simulink model "Kenh_B"  (R2017b)
settings: Solver=FixedStepDiscrete  StartTime=0.0  StopTime=inf  FixedStep=0.0005  RelTol=1e-3  EnableMultiTasking=on
libraries: arduinolib x4, simulink x3
settings Model: SimulationMode=external  ExtModeTrigDuration=2  Creator=Admin  LastModifiedBy=Admin
settings SolverCC: AutoInsertRateTranBlk=on
settings DataIOCC: LimitDataPoints=on
settings OptimizationCC: PassReuseOutputArgsAs=Individual arguments  MaxStackSize=64
settings DebuggingCC: ParameterTunabilityLossMsg=error  AllowSymbolicDim=off  SFUnexpectedBacktrackingDiag=warning  SFNoUnconditionalDefaultTransitionDiag=warning  SFExecutionAtInitializationDiag=none
settings HardwareCC: ProdBitPerInt=16  ProdBitPerPointer=16  ProdBitPerSizeT=16  ProdBitPerPtrDiffT=16  ProdLargestAtomicFloat=None  ProdWordSize=8  ProdHWDeviceType=Atmel->AVR
settings SFSimCC: MATLABDynamicMemAlloc=off
settings RTWCC: SystemTargetFile=ert.tlc  HardwareBoard=Arduino Uno  TLCOptions=-aInlineSetEventsForThisBaseRateFcn=TLC_FALSE -aSuppressMultiTaskScheduler=TLC_FALSE -aRateBasedStepFcn=1  TemplateMakefile=ert_default_tmf  GenerateReport=on  Toolchain=Arduino AVR  BuildConfiguration=Faster Runs  IncludeHyperlinkInReport=on  LaunchReport=on  GenerateTraceInfo=on  GenerateTraceReport=on  GenerateTraceReportSl=on  GenerateTraceReportSf=on  GenerateTraceReportEml=on
settings CodeAppCC: ForceParamTrailComments=on  IgnoreCustomStorageClasses=off  OperatorAnnotations=on  SimulinkDataObjDesc=on  SFDataObjDesc=on  InsertBlockDesc=on
settings ERTTargetCC: SupportContinuousTime=on  SupportVariableSizeSignals=on  ExtMode=on  ExtModeMexArgs='127.0.0.1' 0 17725
settings ConfigComp: CovMetricSettings=dw  CovHtmlReporting=on  CovSaveCumulativeToWorkspaceVar=on  CovSaveSingleToWorkspaceVar=on  CovShowResultsExplorer=off  CovExternalEMLEnable=off  CovSFcnEnable=off

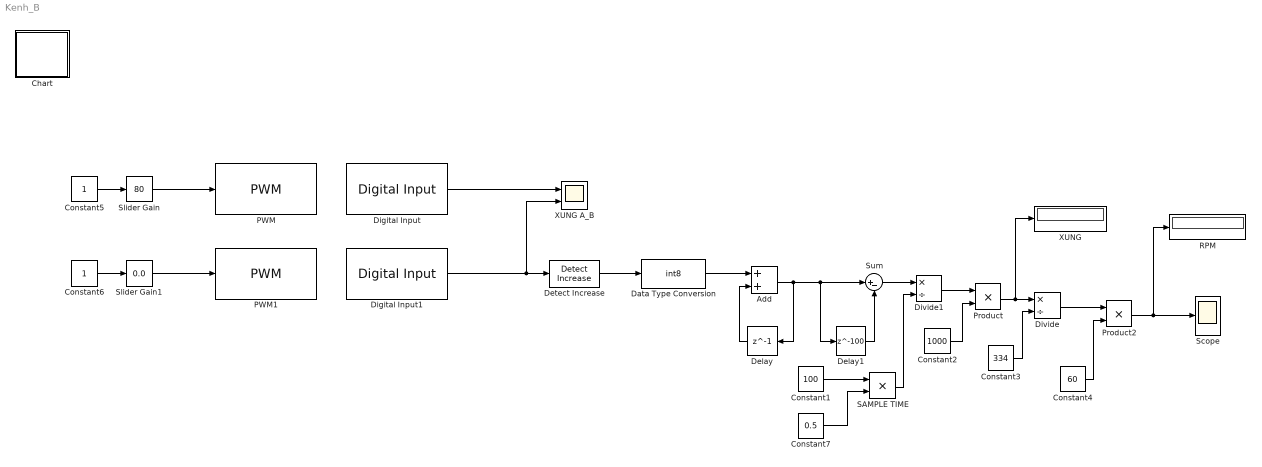
== system Kenh_B ==
  Add : Sum
  Chart : Stateflow chart  TreatAsAtomicUnit=on
  Constant1 : Constant  Value=100
  Constant2 : Constant  Value=1000
  Constant3 : Constant  Value=334
  Constant4 : Constant  Value=60
  Constant5 : Constant
  Constant6 : Constant
  Constant7 : Constant  Value=0.5
  Data Type Conversion : DataTypeConversion  OutDataTypeStr=int8
  Delay : Delay  DelayLength=1  InitialCondition=0
  Delay1 : Delay  DelayLength=100
  Detect Increase : simulink/Logic and Bit Operations/Detect Increase  vinit=0.0  OutDataTypeStr=boolean
  Digital Input : arduinolib/Digital Input  pinNumber=2  sampleTime=-1  blockPlatform=arduino
      settings: SourceProductName=Simulink Support Package for Arduino Hardware
  Digital Input1 : arduinolib/Digital Input  pinNumber=3  sampleTime=-1  blockPlatform=arduino
      settings: SourceProductName=Simulink Support Package for Arduino Hardware
  Divide : Product  Inputs=*/
  Divide1 : Product  Inputs=*/
  PWM : arduinolib/PWM  pinNumber=5  blockPlatform=arduino
  PWM1 : arduinolib/PWM  pinNumber=6  blockPlatform=arduino
  Product : Product
  Product2 : Product
  RPM : Display
  SAMPLE TIME : Product
  Scope : Scope
  Slider Gain : simulink/Math Operations/Slider Gain  gain=80  low=0  high=255
  Slider Gain1 : simulink/Math Operations/Slider Gain  gain=0.0  low=0  high=255
  Sum : Sum  Inputs=|+-
  XUNG : Display
  XUNG A_B : Scope  NumInputPorts=2
  wires:
  Digital Input1/1 -> XUNG A_B/2, Detect Increase/1
  Detect Increase/1 -> Data Type Conversion/1
  Add/1 -> Delay1/1, Sum/1, Delay/1
  Delay/1 -> Add/2
  Delay1/1 -> Sum/2
  Product/1 -> XUNG/1, Divide/1
  Divide/1 -> Product2/1
  Constant3/1 -> Divide/2
  Constant4/1 -> Product2/2
  Constant2/1 -> Product/2
  Slider Gain/1 -> PWM/1
  Constant5/1 -> Slider Gain/1
  Constant6/1 -> Slider Gain1/1
  Slider Gain1/1 -> PWM1/1
  Data Type Conversion/1 -> Add/1
  Digital Input/1 -> XUNG A_B/1
  Product2/1 -> Scope/1, RPM/1
  Sum/1 -> Divide1/1
  Divide1/1 -> Product/1
  SAMPLE TIME/1 -> Divide1/2
  Constant1/1 -> SAMPLE TIME/1
  Constant7/1 -> SAMPLE TIME/2

== stateflow chart Kenh_B/Chart ==
